simulink model "model_2015a"  (R2016a)
settings: Solver=ode4  StartTime=0.0  StopTime=5  FixedStep=0.001  RelTol=1e-3
values from neighbouring files (symbols this model uses):
  b = 0    [fuzzy_cel.m]
  b_nc = [0 0 0]'    [fuzzy_cel.m]    (also in uczenie.m)
  D1 = 1.5    [dane.m]    (also in fuzzy_cel.m; uczenie.m)
  D2 = 1    [dane.m]    (also in fuzzy_cel.m; uczenie.m)
  I1 = 0.002    [dane.m]    (also in fuzzy_cel.m = 0.2; uczenie.m = 0.3)
  I2 = 0.002    [dane.m]    (also in fuzzy_cel.m; uczenie.m)
  J = 1/3*2*0.4^2    (= 0.106666666667)    [dane.m]    (also in fuzzy_cel.m; uczenie.m)
  kd1 = D1    (= 1.5)    [fuzzy_cel.m]    (also in uczenie.m)
  kd2 = D2    (= 1)    [fuzzy_cel.m]    (also in uczenie.m)
  Ke = 10    [dane.m]    (also in fuzzy_cel.m; uczenie.m)
  ki1 = I1    (= 0.2)    [fuzzy_cel.m]    (also in uczenie.m = 0.3)
  ki2 = I2    (= 0.002)    [fuzzy_cel.m]    (also in uczenie.m)
  kp1 = P1    (= 3)    [fuzzy_cel.m]    (also in uczenie.m)
  kp2 = P2    (= 3)    [fuzzy_cel.m]    (also in uczenie.m)
  L = 0.05    [dane.m]    (also in fuzzy_cel.m; uczenie.m)
  P1 = 3    [dane.m]    (also in fuzzy_cel.m; uczenie.m)
  P2 = 3    [dane.m]    (also in fuzzy_cel.m; uczenie.m)
  R = 10    [dane.m]    (also in fuzzy_cel.m; uczenie.m)
  sat_wsp1 = -2.65    [fuzzy_cel.m]    (also in uczenie.m)
  sat_wsp2 = -5.33    [fuzzy_cel.m]    (also in uczenie.m)
  U_g1 = 0.5    [fuzzy_cel.m]    (also in uczenie.m)
  U_g2 = 1    [fuzzy_cel.m]    (also in uczenie.m)
  Umax1 = 0.4    [dane.m]    (also in fuzzy_cel.m = 0.5; uczenie.m = 0.5)
  Umax2 = 1    [dane.m]    (also in fuzzy_cel.m; uczenie.m)
  Umin1 = -Umax1    (= -0.4)    [dane.m]    (also in fuzzy_cel.m = -0.5; uczenie.m = -0.5)
  Umin2 = -Umax2    (= -1)    [dane.m]    (also in fuzzy_cel.m; uczenie.m)
  W = [kd1 kp1 ki1 0 ... (first row only)    [fuzzy_cel.m]    (also in uczenie.m)
  z_max = 1    [fuzzy_cel.m]    (also in uczenie.m)
  z_min = -1    [fuzzy_cel.m]    (also in uczenie.m)
undefined symbols (not defined in the file or in its folder): sigbuilder_block
settings Model: Creator=Student  LastModifiedBy=Maciek
settings DataIOCC: LimitDataPoints=on  SaveFormat=Array
settings HardwareCC: ProdBitPerPointer=32  ProdLargestAtomicFloat=None  ProdIntDivRoundTo=Undefined  ProdEndianess=Unspecified  ProdWordSize=32  ProdHWDeviceType=32-bit Generic
settings ModelReferenceCC: PropagateSignalLabelsOutOfModel=off
settings ConfigComp: CovModelRefEnable=Off

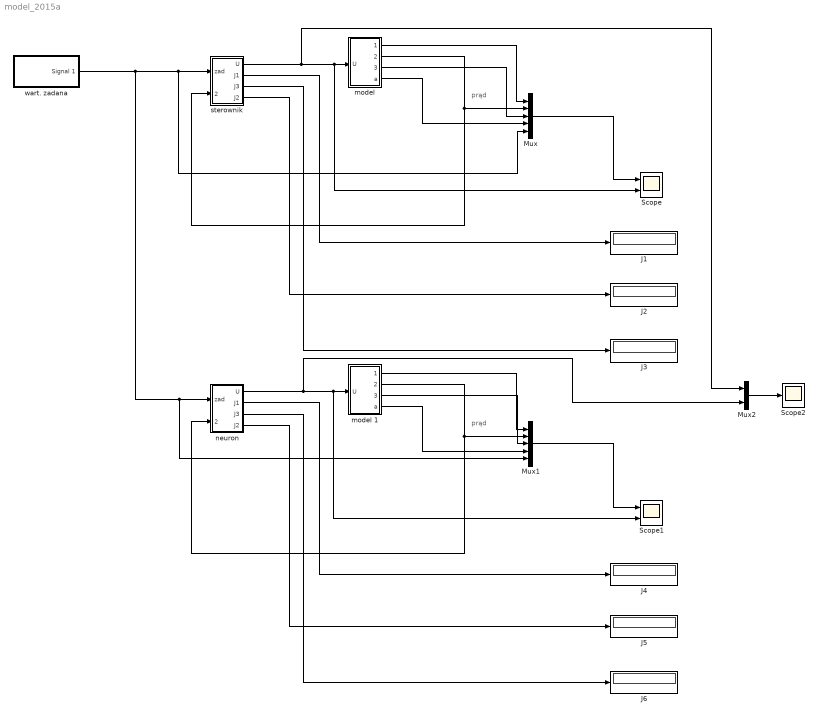
== system model_2015a ==
  note: prąd
  note: prąd
  J{1..6} (6 alike) : Display
  Mux : Mux  Inputs=5
  Mux1 : Mux  Inputs=5
  Mux2 : Mux  Inputs=2
  Scope : Scope  NumInputPorts=2
  Scope1 : Scope  NumInputPorts=2
  Scope2 : Scope
  "model " : Subsystem
  model 1 : Subsystem
  neuron : Subsystem
  sterownik : Subsystem
  wart. zadana : Subsystem  Tag=STV Subsys  LoadFcn=sigbuilder_block('load');  StartFcn=sigbuilder_block('start');  StopFcn=sigbuilder_block('stop');  ClipboardFcn=sigbuilder_block('clipboard');  mask(Sigbuilder block){}
      mask help: Simulink:masks:SigbuilderBlock_MD
      mask init:
      | if ~strcmp(get_param(bdroot(gcbh),'SimulationStatus'),'stopped') tuvar = sigbuilder_block('maskInit'); end
      settings: CopyFcn=sigbuilder_block('copy');  DeleteFcn=sigbuilder_block('delete');  ModelCloseFcn=sigbuilder_block('modelClose');  PreSaveFcn=sigbuilder_block('preSave');  PauseFcn=sigbuilder_block('pause');  ContinueFcn=sigbuilder_block('continue');  NameChangeFcn=sigbuilder_block('namechange');  OpenFcn=sigbuilder_block('open',[437.25 153.75 550.5 359.25 ]);  CloseFcn=sigbuilder_block('close');
      mask Display: plot(0, 0, 100, 100,[2, 2, 32, 32, 2], [68, 8, 8, 68, 68],[32, 2], [38, 38], [32, 19, 2],[53, 60, 44], [32, 17, 17, 2],[16, 16, 31, 31]);txt = getActiveGroup(gcbh);text(2, 100, txt,'verticalAlignment', 'top');
  wires:
  Mux/1 -> Scope/1
  "model "/2(alpha) -> sterownik/2(alpha), Mux/2
  "model "/1(prąd) -> Mux/1
  "model "/3(omega) -> Mux/3
  "model "/4(a) -> Mux/4
  sterownik/1(U) -> Mux2/1, Scope/2, "model "/1(U)
  sterownik/2(J1) -> J1/1
  sterownik/3("J3 ") -> J3/1
  sterownik/4("J2 ") -> J2/1
  Mux1/1 -> Scope1/1
  wart. zadana/1(Signal 1) -> Mux1/5, neuron/1(zad), Mux/5, sterownik/1(zad)
  model 1/2(alpha) -> neuron/2(alpha), Mux1/2
  model 1/1(prąd) -> Mux1/1
  model 1/3(omega) -> Mux1/3
  model 1/4(a) -> Mux1/4
  neuron/1(U) -> Mux2/2, Scope1/2, model 1/1(U)
  neuron/2(J1) -> J4/1
  neuron/3("J3 ") -> J6/1
  neuron/4("J2 ") -> J5/1
  Mux2/1 -> Scope2/1

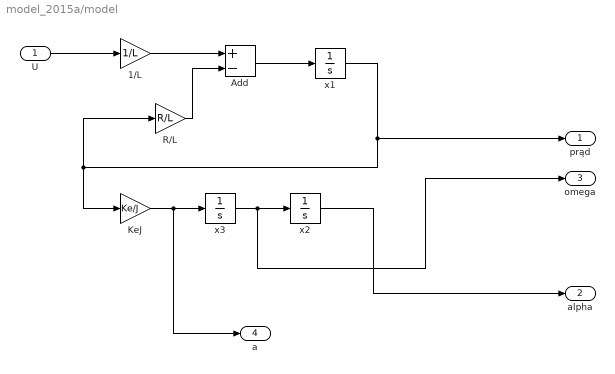
== system model_2015a/model  ==
  U : Inport
  "1/L " : Gain  Gain=1/L
  Add : Sum  Inputs=+-
  KeJ : Gain  Gain=Ke/J
  R/L : Gain  Gain=R/L
  "x1 " : Integrator
  x2 : Integrator  InitialCondition=-1
  "x3 " : Integrator
  prąd : Outport
  alpha : Outport  Port=2
  omega : Outport  Port=3
  a : Outport  Port=4
  wires:
  U/1 -> "1/L "/1
  x2/1 -> alpha/1
  KeJ/1 -> a/1, "x3 "/1
  "x3 "/1 -> omega/1, x2/1
  Add/1 -> "x1 "/1
  "1/L "/1 -> Add/1
  R/L/1 -> Add/2
  "x1 "/1 -> KeJ/1, R/L/1, prąd/1

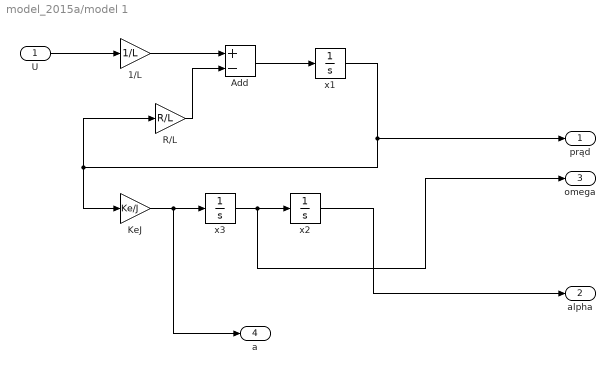
== system model_2015a/model 1 ==
  U : Inport
  "1/L " : Gain  Gain=1/L
  Add : Sum  Inputs=+-
  KeJ : Gain  Gain=Ke/J
  R/L : Gain  Gain=R/L
  "x1 " : Integrator
  x2 : Integrator  InitialCondition=-1
  "x3 " : Integrator
  prąd : Outport
  alpha : Outport  Port=2
  omega : Outport  Port=3
  a : Outport  Port=4
  wires:
  U/1 -> "1/L "/1
  x2/1 -> alpha/1
  KeJ/1 -> a/1, "x3 "/1
  "x3 "/1 -> omega/1, x2/1
  Add/1 -> "x1 "/1
  "1/L "/1 -> Add/1
  R/L/1 -> Add/2
  "x1 "/1 -> KeJ/1, R/L/1, prąd/1

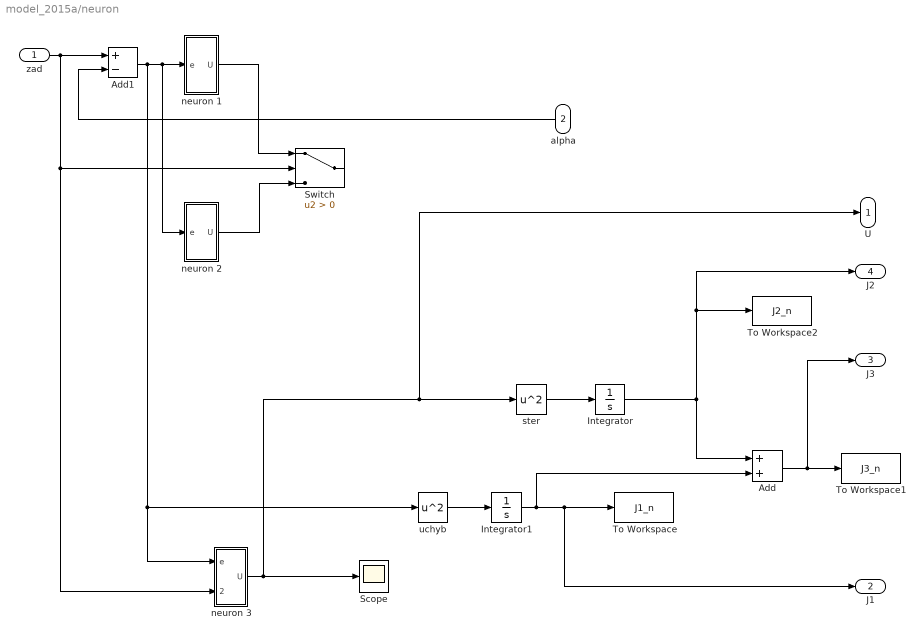
== system model_2015a/neuron ==
  zad : Inport
  alpha : Inport  Port=2
  Add : Sum
  Add1 : Sum  Inputs=+-
  Integrator : Integrator
  Integrator1 : Integrator
  Scope : Scope
  Switch : Switch  Criteria=u2 > Threshold
  To Workspace : ToWorkspace  VariableName=J1_n  SampleTime=-1
      settings: MaxDataPoints=1
  To Workspace1 : ToWorkspace  VariableName=J3_n  SampleTime=-1
      settings: MaxDataPoints=1
  To Workspace2 : ToWorkspace  VariableName=J2_n  SampleTime=-1
      settings: MaxDataPoints=1
  neuron 1 : Subsystem
  neuron 2 : Subsystem
  neuron 3 : Subsystem
  ster : Math  Operator=square  SaturateOnIntegerOverflow=on
  "uchyb " : Math  Operator=square  SaturateOnIntegerOverflow=on
  U : Outport
  J1 : Outport  Port=2
  "J3 " : Outport  Port=3
  "J2 " : Outport  Port=4
  wires:
  neuron 2/1("U ") -> Switch/3
  alpha/1 -> Add1/2
  neuron 1/1("U ") -> Switch/1
  zad/1 -> neuron 3/2(zad), Switch/2, Add1/1
  Add1/1 -> neuron 3/1(e), "uchyb "/1, neuron 2/1(e), neuron 1/1(e)
  ster/1 -> Integrator/1
  "uchyb "/1 -> Integrator1/1
  Integrator1/1 -> Add/2, J1/1, To Workspace/1
  Integrator/1 -> To Workspace2/1, "J2 "/1, Add/1
  Add/1 -> "J3 "/1, To Workspace1/1
  neuron 3/1("U ") -> U/1, ster/1, Scope/1

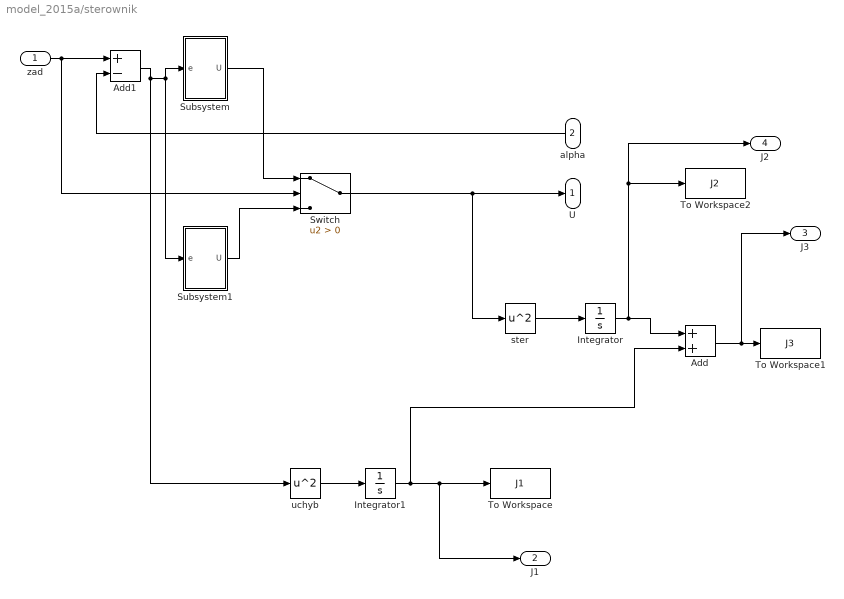
== system model_2015a/sterownik ==
  zad : Inport
  alpha : Inport  Port=2
  Add : Sum
  Add1 : Sum  Inputs=+-
  Integrator : Integrator
  Integrator1 : Integrator
  Subsystem : Subsystem
  Subsystem1 : Subsystem
  Switch : Switch  Criteria=u2 > Threshold
  To Workspace : ToWorkspace  VariableName=J1  SampleTime=-1
      settings: MaxDataPoints=1
  To Workspace1 : ToWorkspace  VariableName=J3  SampleTime=-1
      settings: MaxDataPoints=1
  To Workspace2 : ToWorkspace  VariableName=J2  SampleTime=-1
      settings: MaxDataPoints=1
  ster : Math  Operator=square  SaturateOnIntegerOverflow=on
  "uchyb " : Math  Operator=square  SaturateOnIntegerOverflow=on
  U : Outport
  J1 : Outport  Port=2
  "J3 " : Outport  Port=3
  "J2 " : Outport  Port=4
  wires:
  Subsystem1/1(U) -> Switch/3
  Switch/1 -> ster/1, U/1
  alpha/1 -> Add1/2
  Subsystem/1(U) -> Switch/1
  zad/1 -> Switch/2, Add1/1
  Add1/1 -> Subsystem1/1(e), Subsystem/1(e), "uchyb "/1
  ster/1 -> Integrator/1
  "uchyb "/1 -> Integrator1/1
  Integrator1/1 -> Add/2, J1/1, To Workspace/1
  Integrator/1 -> To Workspace2/1, "J2 "/1, Add/1
  Add/1 -> "J3 "/1, To Workspace1/1

== system model_2015a/wart. zadana ==
  Demux : Demux  Tag=STV Demux  Outputs=1
  FromWs : FromWorkspace  Tag=STV FromWs  VariableName=tuvar  SampleTime=0
      SigBuilderData=|
      | common.afterFinalStr = 'Extrapolate'
      | common.sampleTime = 0
      | dataSet.timeRange = [0 10]
      | dataSet.name = 'Group 1'
      | sbobj.Groups.Name = 'Group 1'
      | sbobj.Groups.Signals.Name = 'Signal 1'
      | sbobj.Groups.Signals.XData = [0 3 3 5 5 8 8 10]
      | sbobj.Groups.Signals.YData = [1 1 -1 -1 1 1 -1 -1]
  Signal 1 : Outport  Tag=STV Outport
  wires:
  FromWs/1 -> Demux/1
  Demux/1 -> Signal 1/1

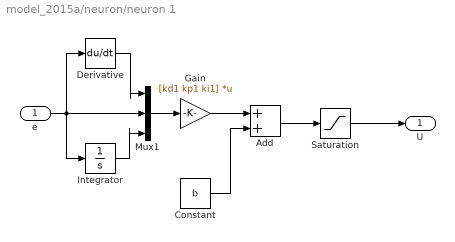
== system model_2015a/neuron/neuron 1 ==
  e : Inport
  Add : Sum
  Constant : Constant  Value=b
  Derivative : Derivative
  Gain : Gain  Gain=[kd1 kp1 ki1]  Multiplication=Matrix(K*u) (u vector)
  Integrator : Integrator
  Mux1 : Mux  Inputs=3
  Saturation : Saturate  UpperLimit=Umax1  LowerLimit=Umin1
  "U " : Outport
  wires:
  Integrator/1 -> Mux1/3
  e/1 -> Integrator/1, Mux1/2, Derivative/1
  Derivative/1 -> Mux1/1
  Gain/1 -> Add/1
  Constant/1 -> Add/2
  Add/1 -> Saturation/1
  Mux1/1 -> Gain/1
  Saturation/1 -> "U "/1

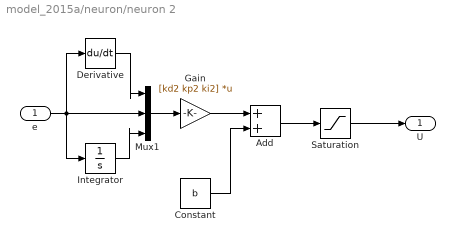
== system model_2015a/neuron/neuron 2 ==
  e : Inport
  Add : Sum
  Constant : Constant  Value=b
  Derivative : Derivative
  Gain : Gain  Gain=[kd2 kp2 ki2]  Multiplication=Matrix(K*u) (u vector)
  Integrator : Integrator
  Mux1 : Mux  Inputs=3
  Saturation : Saturate  UpperLimit=Umax2  LowerLimit=Umin2
  "U " : Outport
  wires:
  Integrator/1 -> Mux1/3
  e/1 -> Integrator/1, Mux1/2, Derivative/1
  Derivative/1 -> Mux1/1
  Gain/1 -> Add/1
  Constant/1 -> Add/2
  Add/1 -> Saturation/1
  Mux1/1 -> Gain/1
  Saturation/1 -> "U "/1

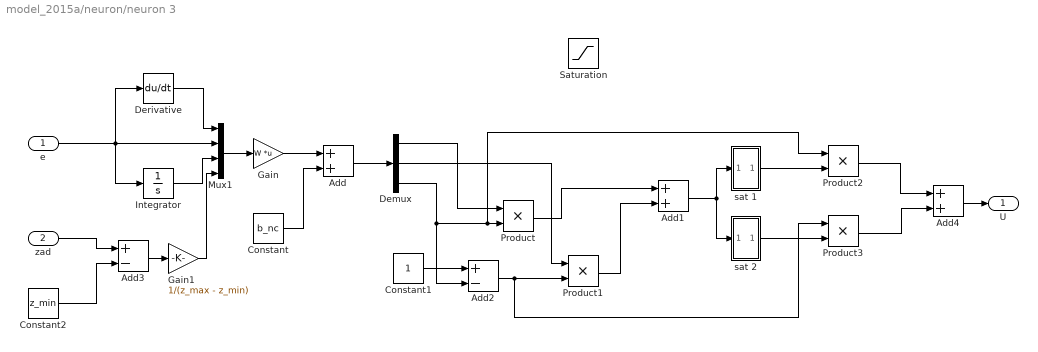
== system model_2015a/neuron/neuron 3 ==
  e : Inport
  zad : Inport  Port=2
  Add : Sum
  Add1 : Sum
  Add2 : Sum  Inputs=+-
  Add3 : Sum  Inputs=+-
  Add4 : Sum
  Constant : Constant  Value=b_nc
  Constant1 : Constant
  Constant2 : Constant  Value=z_min
  Demux : Demux  Outputs=3
  Derivative : Derivative
  Gain : Gain  Gain=W  Multiplication=Matrix(K*u) (u vector)
  Gain1 : Gain  Gain=1/(z_max - z_min)
  Integrator : Integrator
  Mux1 : Mux
  Product{,1..3} (4 alike) : Product
  Saturation : Saturate  UpperLimit=Umax1  LowerLimit=Umin1
  sat 1 : Subsystem
  sat 2 : Subsystem
  "U " : Outport
  wires:
  Integrator/1 -> Mux1/3
  e/1 -> Integrator/1, Derivative/1, Mux1/2
  Derivative/1 -> Mux1/1
  Gain/1 -> Add/1
  Constant/1 -> Add/2
  Mux1/1 -> Gain/1
  Add1/1 -> sat 2/1(in), sat 1/1(in)
  Add/1 -> Demux/1
  Demux/2 -> Product1/1
  Demux/1 -> Product/1
  Demux/3 -> Add2/2, Product2/1, Product/2
  Product/1 -> Add1/1
  Constant1/1 -> Add2/1
  Add2/1 -> Product3/1, Product1/2
  Product1/1 -> Add1/2
  Add3/1 -> Gain1/1
  zad/1 -> Add3/1
  Constant2/1 -> Add3/2
  sat 1/1(u) -> Product2/2
  sat 2/1(u) -> Product3/2
  Product2/1 -> Add4/1
  Product3/1 -> Add4/2
  Add4/1 -> "U "/1
  Gain1/1 -> Mux1/4

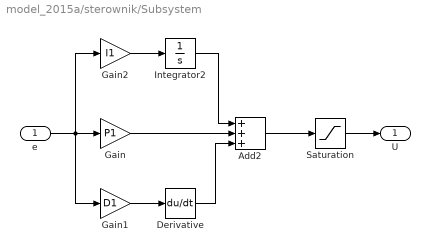
== system model_2015a/sterownik/Subsystem ==
  e : Inport
  Add2 : Sum  Inputs=+++
  Derivative : Derivative
  Gain : Gain  Gain=P1
  Gain1 : Gain  Gain=D1
  Gain2 : Gain  Gain=I1
  Integrator2 : Integrator
  Saturation : Saturate  UpperLimit=Umax1  LowerLimit=Umin1
  U : Outport
  wires:
  Derivative/1 -> Add2/3
  e/1 -> Gain1/1, Gain/1, Gain2/1
  Integrator2/1 -> Add2/1
  Add2/1 -> Saturation/1
  Gain/1 -> Add2/2
  Gain1/1 -> Derivative/1
  Gain2/1 -> Integrator2/1
  Saturation/1 -> U/1

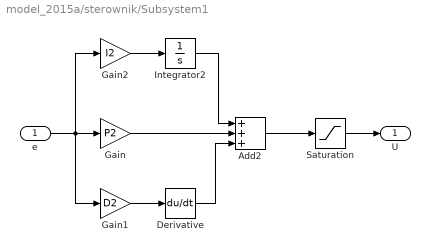
== system model_2015a/sterownik/Subsystem1 ==
  e : Inport
  Add2 : Sum  Inputs=+++
  Derivative : Derivative
  Gain : Gain  Gain=P2
  Gain1 : Gain  Gain=D2
  Gain2 : Gain  Gain=I2
  Integrator2 : Integrator
  Saturation : Saturate  UpperLimit=Umax2  LowerLimit=Umin2
  U : Outport
  wires:
  Derivative/1 -> Add2/3
  e/1 -> Gain1/1, Gain/1, Gain2/1
  Integrator2/1 -> Add2/1
  Add2/1 -> Saturation/1
  Gain/1 -> Add2/2
  Gain1/1 -> Derivative/1
  Gain2/1 -> Integrator2/1
  Saturation/1 -> U/1

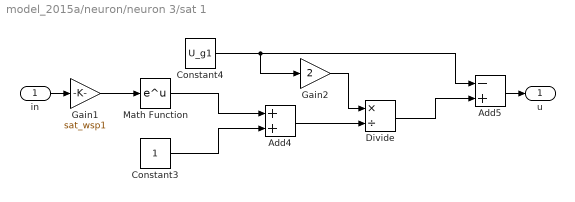
== system model_2015a/neuron/neuron 3/sat 1 ==
  in : Inport
  Add4 : Sum
  Add5 : Sum  Inputs=-+
  Constant3 : Constant
  Constant4 : Constant  Value=U_g1
  Divide : Product  Inputs=*/
  Gain1 : Gain  Gain=sat_wsp1
  Gain2 : Gain  Gain=2
  Math Function : Math  SaturateOnIntegerOverflow=on
  u : Outport
  wires:
  Divide/1 -> Add5/2
  Math Function/1 -> Add4/1
  Constant4/1 -> Gain2/1, Add5/1
  Gain1/1 -> Math Function/1
  Gain2/1 -> Divide/1
  Add4/1 -> Divide/2
  Constant3/1 -> Add4/2
  in/1 -> Gain1/1
  Add5/1 -> u/1

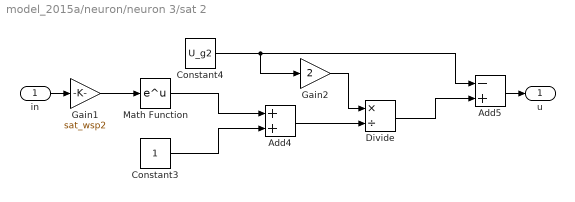
== system model_2015a/neuron/neuron 3/sat 2 ==
  in : Inport
  Add4 : Sum
  Add5 : Sum  Inputs=-+
  Constant3 : Constant
  Constant4 : Constant  Value=U_g2
  Divide : Product  Inputs=*/
  Gain1 : Gain  Gain=sat_wsp2
  Gain2 : Gain  Gain=2
  Math Function : Math  SaturateOnIntegerOverflow=on
  u : Outport
  wires:
  Divide/1 -> Add5/2
  Math Function/1 -> Add4/1
  Constant4/1 -> Gain2/1, Add5/1
  Gain1/1 -> Math Function/1
  Gain2/1 -> Divide/1
  Add4/1 -> Divide/2
  Constant3/1 -> Add4/2
  in/1 -> Gain1/1
  Add5/1 -> u/1
